simulink model "PID_fuzzy"  (R2017a)
settings: Solver=VariableStepAuto  StartTime=0.0  StopTime=5.0  RelTol=1e-3
undefined symbols (not defined in the file or in its folder): f2
libraries: fuzblock x1
settings Model: Creator=Lenovo  LastModifiedBy=Lenovo
settings SolverCC: ZeroCrossAlgorithm=Adaptive

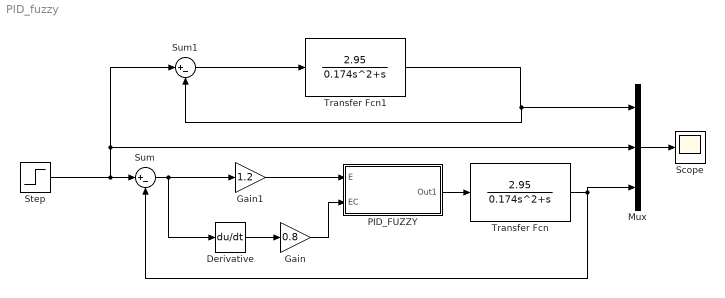
== system PID_fuzzy ==
  Derivative : Derivative
  Gain : Gain  Gain=0.8
  Gain1 : Gain  Gain=1.2
  Mux : Mux  Inputs=3
  PID_FUZZY : Subsystem
  Scope : Scope
  Step : Step  After=1500  SampleTime=0.01
  Sum : Sum  Inputs=|+-
  Sum1 : Sum  Inputs=|+-
  Transfer Fcn : TransferFcn  Numerator=[2.95]  Denominator=[0.174 1 0]
  Transfer Fcn1 : TransferFcn  Numerator=[2.95]  Denominator=[0.174 1 0]
  wires:
  Step/1 -> Sum1/1, Mux/2, Sum/1
  Sum/1 -> Derivative/1, Gain1/1
  Transfer Fcn/1 -> Sum/2, Mux/3
  Mux/1 -> Scope/1
  Transfer Fcn1/1 -> Sum1/2, Mux/1
  Sum1/1 -> Transfer Fcn1/1
  PID_FUZZY/1(Out1) -> Transfer Fcn/1
  Derivative/1 -> Gain/1
  Gain/1 -> PID_FUZZY/2(EC)
  Gain1/1 -> PID_FUZZY/1(E)

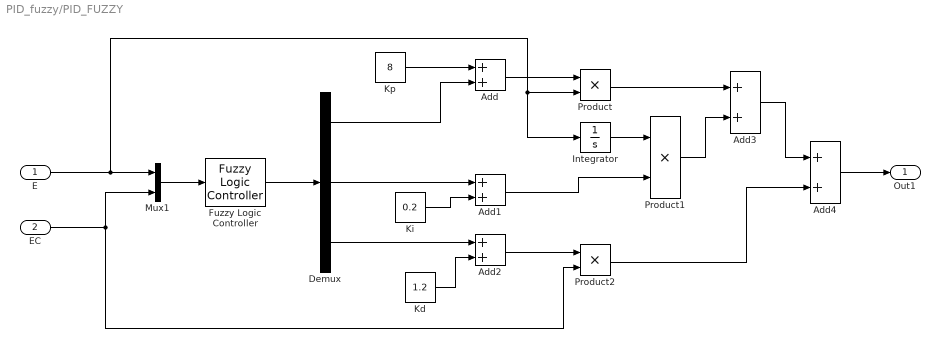
== system PID_fuzzy/PID_FUZZY ==
  E : Inport
  EC : Inport  Port=2
  Add{,1..4} (5 alike) : Sum
  Demux : Demux  Outputs=3
  Fuzzy Logic Controller : fuzblock/Fuzzy Logic  Controller  fis=[f2]
  Integrator : Integrator
  Kd : Constant  Value=1.2
  Ki : Constant  Value=0.2
  Kp : Constant  Value=8
  Mux1 : Mux  Inputs=2
  Product : Product
  Product1 : Product
  Product2 : Product
  Out1 : Outport
  wires:
  Mux1/1 -> Fuzzy Logic Controller/1
  Ki/1 -> Add1/2
  Kp/1 -> Add/1
  EC/1 -> Product2/2, Mux1/2
  Fuzzy Logic Controller/1 -> Demux/1
  E/1 -> Integrator/1, Product/2, Mux1/1
  Add/1 -> Product/1
  Demux/2 -> Add1/1
  Demux/1 -> Add/2
  Product2/1 -> Add4/2
  Add4/1 -> Out1/1
  Add3/1 -> Add4/1
  Demux/3 -> Add2/1
  Integrator/1 -> Product1/1
  Add2/1 -> Product2/1
  Kd/1 -> Add2/2
  Add1/1 -> Product1/2
  Product/1 -> Add3/1
  Product1/1 -> Add3/2
